simulink model "rom_waam"  (R2021a)
settings: Solver=VariableStepAuto  StartTime=0.0  StopTime=10  FixedStep=1e-3  RelTol=1e-3
InitFcn:
  | net = load('./net.mat').net
libraries: simulink x1, deeplib x1
settings Model: Creator=giulio  LastModifiedBy=giulio

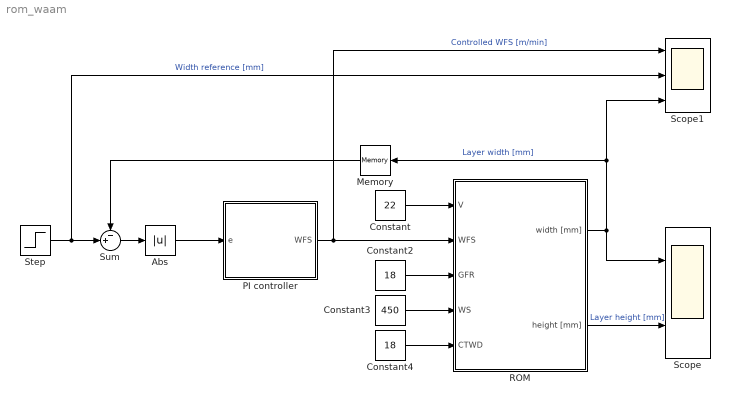
== system rom_waam ==
  Abs : Abs
  Constant : Constant  Value=22
  Constant2 : Constant  Value=18
  Constant3 : Constant  Value=450
  Constant4 : Constant  Value=18
  Memory : Memory
  PI controller : Subsystem
  ROM : Subsystem
  Scope : Scope  NumInputPorts=2
  Scope1 : Scope  NumInputPorts=3
  Step : Step  Time=5  Before=4  After=6  SampleTime=0
  Sum : Sum  Inputs=-+|
  wires:
  Constant/1 -> ROM/1(V)
  PI controller/1(WFS) -> Scope1/1, ROM/2(WFS)  "Controlled WFS [m/min]"
  Constant2/1 -> ROM/3(GFR)
  ROM/2(height [mm]) -> Scope/2  "Layer height [mm]"
  Step/1 -> Scope1/2, Sum/2  "Width reference [mm]"
  ROM/1(width [mm]) -> Memory/1, Scope1/3, Scope/1  "Layer width [mm]"
  Constant4/1 -> ROM/5(CTWD)
  Memory/1 -> Sum/1
  Sum/1 -> Abs/1
  Abs/1 -> PI controller/1(e)
  Constant3/1 -> ROM/4(WS)

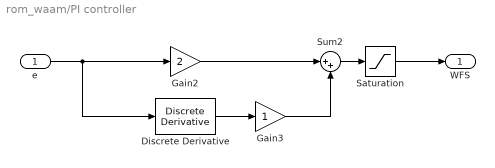
== system rom_waam/PI controller ==
  e : Inport
  Discrete Derivative : simulink/Discrete/Discrete Derivative  gainval=1.0  ICPrevScaledInput=0.0  OutMin=[]  OutMax=[]  OutDataType=fixdt(1, 16)  OutScaling=2^-10  DoSatur=off
  Gain2 : Gain  Gain=2
  Gain3 : Gain
  Saturation : Saturate  UpperLimit=10  LowerLimit=2
  Sum2 : Sum  Inputs=|++
  WFS : Outport
  wires:
  Sum2/1 -> Saturation/1
  e/1 -> Gain2/1, Discrete Derivative/1
  Discrete Derivative/1 -> Gain3/1
  Gain3/1 -> Sum2/2
  Gain2/1 -> Sum2/1
  Saturation/1 -> WFS/1

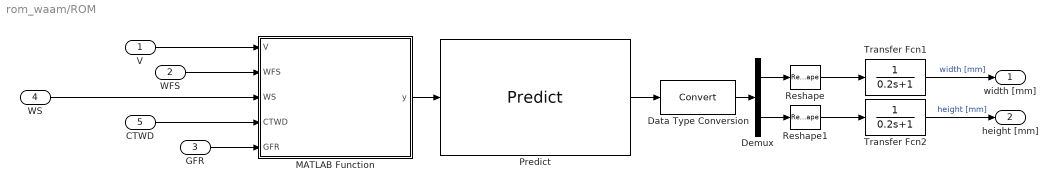
== system rom_waam/ROM ==
  V : Inport
  WFS : Inport  Port=2
  GFR : Inport  Port=3
  WS : Inport  Port=4
  CTWD : Inport  Port=5
  Data Type Conversion : DataTypeConversion
  Demux : Demux  Outputs=2
  MATLAB Function : MATLAB Function  TreatAsAtomicUnit=on
  Predict : deeplib/Predict  Network=Network from MAT-file  NetworkFunction=squeezenet  NetworkFilePath=/home/giulio/Desktop/Math_AI_web/Mathworks-UniNA-AI/waam-rom/net.mat  MiniBatchSize=128  InputDataFormats={ '', '' }  Predictions=on  Activations={}  ForceInterpretedSim=off  EnableDLNetwork=on
      settings: SourceProductBaseCode=NN
  Reshape : Reshape  OutputDimensionality=Customize  OutputDimensions=1
  Reshape1 : Reshape  OutputDimensionality=Customize  OutputDimensions=1
  Transfer Fcn1 : TransferFcn  Denominator=[0.2 1]
  Transfer Fcn2 : TransferFcn  Denominator=[0.2 1]
  width [mm] : Outport
  height [mm] : Outport  Port=2
  wires:
  Data Type Conversion/1 -> Demux/1
  Demux/1 -> Reshape/1
  Transfer Fcn1/1 -> width [mm]/1  "width [mm]"
  WS/1 -> MATLAB Function/3(WS)
  MATLAB Function/1(y) -> Predict/1
  Transfer Fcn2/1 -> height [mm]/1  "height [mm]"
  Predict/1 -> Data Type Conversion/1
  WFS/1 -> MATLAB Function/2(WFS)
  CTWD/1 -> MATLAB Function/4(CTWD)
  Demux/2 -> Reshape1/1
  V/1 -> MATLAB Function/1(V)
  GFR/1 -> MATLAB Function/5(GFR)
  Reshape/1 -> Transfer Fcn1/1
  Reshape1/1 -> Transfer Fcn2/1

== matlab function rom_waam/ROM/MATLAB Function ==
  data: V input; y output; WFS input; WS input; CTWD input; GFR input
function y = convert_input(V, WFS, WS, CTWD, GFR)

y = [V, WFS, WS, CTWD, GFR];
